simulink library "Lib_Vol_FlowStart_TMATS_org"  (Simulink 10.0)
settings: Solver=ode45  StartTime=0.0  StopTime=10.0  RelTol=1e-3  EnableMultiTasking=on
undefined symbols (not defined in the file): Fluid
libraries: Lib_Vol_PropLookup_TMATS x1
Description:
  | Thomas Modules
settings Model: Creator=jwchapm2  LastModifiedBy=bhisma

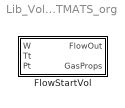
== system Lib_Vol_FlowStart_TMATS_org ==
  FlowStartVol : Subsystem  mask(T-MATS: FlowStart Library Block){TtVec_M=Fluid.Vec.Tt, PtVec_M=Fluid.Vec.Pt, htVec_M=Fluid.Vec.ht, sVec_M=Fluid.Vec.s, htArray_M=Fluid.Array.ht, TtArray_M=Fluid.Array.Tt, sArray_M=Fluid.Array.s, rhoArray_M=Fluid.Array.rho, muArray_M=Fluid.Array.mu, CpArray_M=Fluid.Array.Cp, CvArray_M=Fluid.Array.Cv, CvArray_M_copy=Fluid.Array.u, Rval_M=Fluid.Array.R}
      mask prompts: TtVec_M "TtVec_M - Temperature vector"; PtVec_M "PtVec_M - Pressure vector"; htVec_M "htVec_M - Enthalpy vector"; sVec_M "sVec_M - Entropy vector"; htArray_M "htArray_M - Enthalpy Array f(Tt,Pt)"; TtArray_M "TtArray_M - Temperature Array f(ht,Pt)"; sArray_M "sArray_M - Entropy Array f(ht,Pt)"; rhoArray_M "rhoArray_M - Density Array f(ht,Pt)"; muArray_M "muArray_M - Viscosity Array f(ht,Pt)"; CpArray_M "CpArray_M - Pressure specific heat Array f(ht,Pt)"; CvArray_M "CvArray_M - Volume specific heat Array f(ht,Pt)"; CvArray_M_copy "uArray_M - Internal energy Array f(ht,Pt)"; Rval_M "Rval_M - R value"
      mask help: This block simulates the initialization of fluid properties through a lookup table based on total pressure and temperature.
      mask Help: web(which('Vol_TMATS FlowStart.html'),'-helpbrowser')

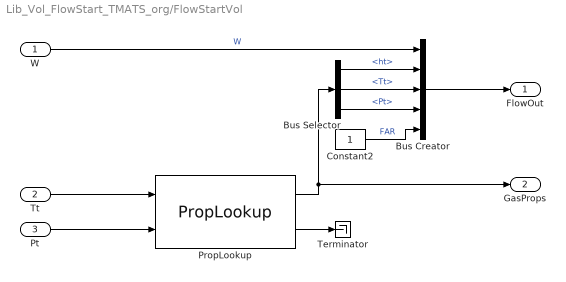
== system Lib_Vol_FlowStart_TMATS_org/FlowStartVol ==
  W : Inport
  "Tt " : Inport  Port=2
  Pt : Inport  Port=3
  Bus Creator : BusCreator  Inputs=5
  Bus Selector : BusSelector  OutputSignals=ht,Tt,Pt
  Constant2 : Constant
  PropLookup : Lib_Vol_PropLookup_TMATS/PropLookup  case_M='Tt'  propg_M=0  htg_M=0  htVec_M=htVec_M  PtVec_M=PtVec_M  TtVec_M=TtVec_M  sVec_M=sVec_M  htArray_M=htArray_M  rhoArray_M=rhoArray_M  uArray_M=ones(length(htVec_M), length(PtVec_M))'  sArray_M=sArray_M  muArray_M=muArray_M  ThArray_M=TtArray_M  CvArray_M=CvArray_M  CpArray_M=CpArray_M  kArray_M=ones(length(htVec_M), length(PtVec_M))'  TsArray_M=ones(length(sVec_M), length(PtVec_M))'  hsArray_M=ones(length(sVec_M), length(PtVec_M))'  Rval_M=Rval_M
  Terminator : Terminator
  FlowOut : Outport
  GasProps : Outport  Port=2
  wires:
  Bus Creator/1 -> FlowOut/1
  W/1 -> Bus Creator/1  "W"
  Pt/1 -> PropLookup/2
  "Tt "/1 -> PropLookup/1
  PropLookup/2 -> Terminator/1
  PropLookup/1 -> GasProps/1, Bus Selector/1
  Bus Selector/3 -> Bus Creator/4  "<Pt>"
  Bus Selector/2 -> Bus Creator/3  "<Tt>"
  Bus Selector/1 -> Bus Creator/2  "<ht>"
  Constant2/1 -> Bus Creator/5  "FAR"
